simulink model "TargetPointTrackingRobotEnv"  (R2025a)
settings: Solver=VariableStepAuto  StartTime=0.0  StopTime=10.0  RelTol=1e-3
values from neighbouring files (symbols this model uses):
  x0 = cos(t1)*R    [TargetPointTrackingRobotResetFcn.m]
  y0 = sin(t1)*R    [TargetPointTrackingRobotResetFcn.m]
undefined symbols (not defined in the file or in its folder): theta0
libraries: rllib x1
settings Model: Creator=ex  LastModifiedBy=ex

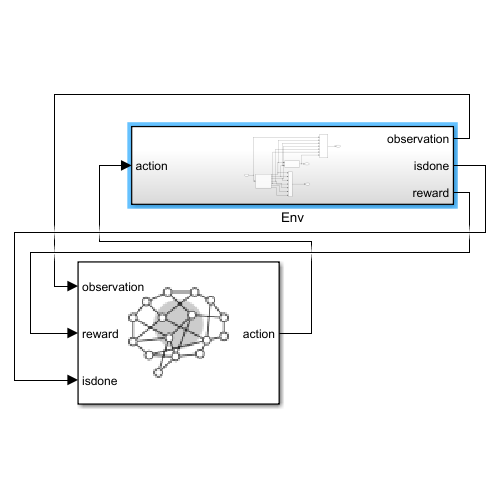
[thumbnail: Simulink's stored preview of the top-level diagram]
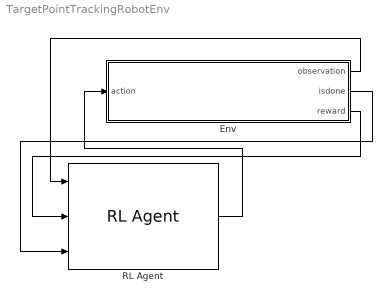
== system TargetPointTrackingRobotEnv ==
  Env : Subsystem
  RL Agent : rllib/RL Agent  Agent=agent  ExternalActionAsInput=off  ProvideLastAction=off  ProvideCumRwd=off  TreatAsDirectFeedthrough=on  UseStrictObservationDataTypes=off
  wires:
  RL Agent/1 -> Env/1(action)
  Env/2(isdone) -> RL Agent/3
  Env/3(reward) -> RL Agent/2
  Env/1(observation) -> RL Agent/1

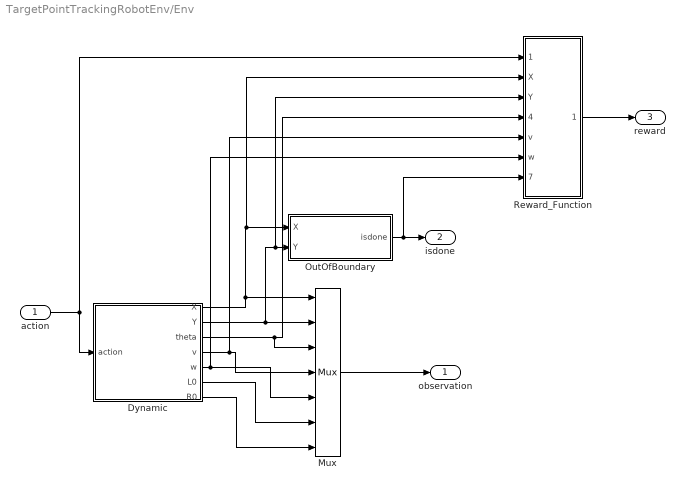
== system TargetPointTrackingRobotEnv/Env ==
  action : Inport
  Dynamic : Subsystem
  Mux : Mux  Inputs=7
  OutOfBoundary : Subsystem
  Reward_Function : Subsystem
  observation : Outport
  isdone : Outport  Port=2
  reward : Outport  Port=3
  wires:
  action/1 -> Reward_Function/1(action), Dynamic/1(action)
  Dynamic/1(X) -> Reward_Function/2(X), OutOfBoundary/1(X), Mux/1
  Dynamic/2(Y) -> Reward_Function/3(Y), OutOfBoundary/2(Y), Mux/2
  Dynamic/3(theta) -> Reward_Function/4(theta), Mux/3
  Mux/1 -> observation/1
  OutOfBoundary/1(isdone) -> Reward_Function/7(isdone), isdone/1
  Reward_Function/1(Reward) -> reward/1
  Dynamic/4(v) -> Reward_Function/5(v), Mux/4
  Dynamic/5(w) -> Reward_Function/6(w), Mux/5
  Dynamic/6(L0) -> Mux/6
  Dynamic/7(R0) -> Mux/7

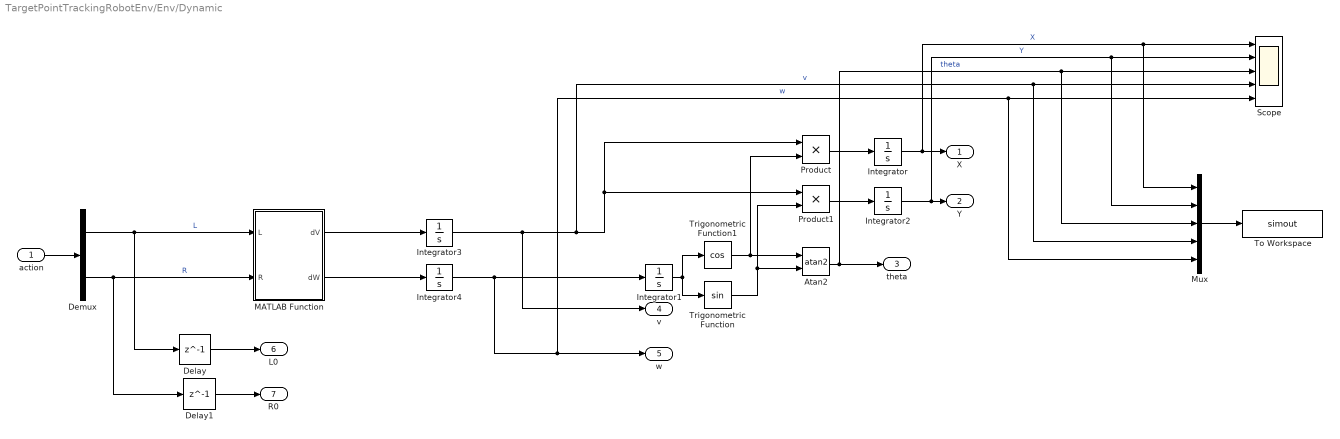
== system TargetPointTrackingRobotEnv/Env/Dynamic ==
  action : Inport
  Atan2 : Trigonometry  Operator=atan2
  Delay : Delay  DelayLength=1  InitialCondition=0
  Delay1 : Delay  DelayLength=1  InitialCondition=0
  Demux : Demux  Outputs=2
  Integrator : Integrator  InitialCondition=x0
  Integrator1 : Integrator  InitialCondition=theta0
  Integrator2 : Integrator  InitialCondition=y0
  Integrator3 : Integrator
  Integrator4 : Integrator
  MATLAB Function : MATLAB Function  TreatAsAtomicUnit=on
  Mux : Mux  Inputs=5
  Product : Product
  Product1 : Product
  Scope : Scope  NumInputPorts=5
      settings: ActiveDisplayYMinimum=-29.512641911410267  ActiveDisplayYMaximum=36.2250173593529
  To Workspace : ToWorkspace  VariableName=simout  SaveFormat=Structure With Time  SampleTime=-1
  Trigonometric Function : Trigonometry
  Trigonometric Function1 : Trigonometry  Operator=cos
  X : Outport
  Y : Outport  Port=2
  theta : Outport  Port=3
  v : Outport  Port=4
  w : Outport  Port=5
  L0 : Outport  Port=6
  R0 : Outport  Port=7
  wires:
  Trigonometric Function1/1 -> Product/2, Atan2/1
  Trigonometric Function/1 -> Product1/2, Atan2/2
  action/1 -> Demux/1
  Integrator1/1 -> Trigonometric Function1/1, Trigonometric Function/1
  Product1/1 -> Integrator2/1
  Integrator2/1 -> Mux/2, Scope/2, Y/1  "Y"
  Product/1 -> Integrator/1
  Integrator/1 -> Mux/1, Scope/1, X/1  "X"
  Atan2/1 -> theta/1, Mux/3, Scope/3  "theta"
  Demux/1 -> Delay/1, MATLAB Function/1(L)  "L"
  Demux/2 -> Delay1/1, MATLAB Function/2(R)  "R"
  MATLAB Function/1(dV) -> Integrator3/1
  MATLAB Function/2(dW) -> Integrator4/1
  Integrator4/1 -> Mux/5, Scope/5, w/1, Integrator1/1  "w"
  Integrator3/1 -> v/1, Mux/4, Scope/4, Product1/1, Product/1  "v"
  Delay/1 -> L0/1
  Delay1/1 -> R0/1
  Mux/1 -> To Workspace/1

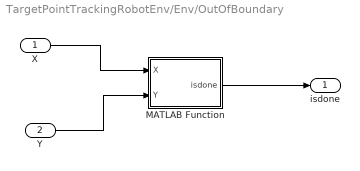
== system TargetPointTrackingRobotEnv/Env/OutOfBoundary ==
  X : Inport
  Y : Inport  Port=2
  MATLAB Function : MATLAB Function  TreatAsAtomicUnit=on
  isdone : Outport
  wires:
  X/1 -> MATLAB Function/1(X)
  Y/1 -> MATLAB Function/2(Y)
  MATLAB Function/1(isdone) -> isdone/1

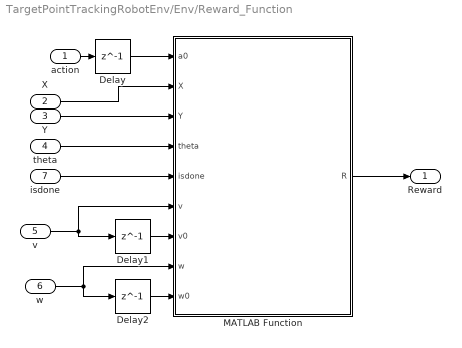
== system TargetPointTrackingRobotEnv/Env/Reward_Function ==
  action : Inport
  X : Inport  Port=2
  Y : Inport  Port=3
  theta : Inport  Port=4
  v : Inport  Port=5
  w : Inport  Port=6
  isdone : Inport  Port=7
  Delay : Delay  DelayLength=1  InitialCondition=0
  Delay1 : Delay  DelayLength=1  InitialCondition=0
  Delay2 : Delay  DelayLength=1  InitialCondition=0
  MATLAB Function : MATLAB Function  TreatAsAtomicUnit=on
  Reward : Outport
  wires:
  MATLAB Function/1(R) -> Reward/1
  action/1 -> Delay/1
  X/1 -> MATLAB Function/2(X)
  Y/1 -> MATLAB Function/3(Y)
  theta/1 -> MATLAB Function/4(theta)
  Delay/1 -> MATLAB Function/1(a0)
  v/1 -> MATLAB Function/6(v), Delay1/1
  w/1 -> Delay2/1, MATLAB Function/8(w)
  Delay1/1 -> MATLAB Function/7(v0)
  Delay2/1 -> MATLAB Function/9(w0)
  isdone/1 -> MATLAB Function/5(isdone)

== matlab function TargetPointTrackingRobotEnv/Env/OutOfBoundary/MATLAB Function ==
  data: X input; isdone output; Y input
function isdone = fcn(X, Y)

boundary = 20;
isdone = false;
if abs(X) > boundary || abs(Y) > boundary
    isdone = true;
end

== matlab function TargetPointTrackingRobotEnv/Env/Reward_Function/MATLAB Function ==
  data: a0 input; R output; X input; Y input; theta input; isdone input; v input; v0 input; w input; w0 input
function R = fcn(a0, X, Y, theta, isdone, v, v0, w, w0)

tarX = 0;
tarY = 0;
tarTheta = 0;

%Penalty of out of boundary
boundaryPenalty = 0;
if isdone 
    boundaryPenalty = -100;
end

% Reward for reaching near target position and orientation
distanceToTarget = 3*(X - tarX)^2 + 3*(Y - tarY)^2 ;
posR = 10 / (1 + 3 * distanceToTarget);
posP = -0.01 * distanceToTarget;
tarAngleR = 0;
if distanceToTarget < 0.5 && abs(tarTheta - theta) < 0.5
    tarAngleR = 5;
end


% penalty for largest movement change
actionSmoothnessR = -0.03 * (v0 - v)^2;

% penalty for sharp turning
deltaW = abs(w0 - w); 
sharpTuringP = -0.05 * deltaW^2;


%penalty for large anglur velocity
if abs(w) > 1.0
    wPenalty = -0.01 * w^2;   
else
    wPenalty = 0;
end

%penalty for larget total torque or largest torque difference
totalTorPenalty = -0.01 * sum(a0.^2);  
diffTorPenalty = -0.01 * (a0(1) - a0(2))^2;

R = posR + posP + tarAngleR + boundaryPenalty + sharpTuringP + actionSmoothnessR + totalTorPenalty + diffTorPenalty + wPenalty;

== matlab function TargetPointTrackingRobotEnv/Env/Dynamic/MATLAB Function ==
  data: L input; dV output; R input; dW output
function [dV, dW] = fcn(L, R)
    % Robot parameters 
    m = 10;      % mass (kg)
    I = 5;       % moment of inertia (kg*m^2)
    r = 0.1;     % wheel radius (m)
    Ri = 0.2;    % distance for each wheel to center (m)

    % Compute linear and angular acceleration
    dV = (1 / (m * r)) * (L + R);
    dW = (2 * Ri / (I * r)) * (L - R);
end
